simulink model "STOICAL_example_1"  (R2015b)
settings: Solver=ode4  StartTime=0.0  StopTime=1  FixedStep=50E-6  RelTol=1e-3
model workspace (MAT data in the model file):
  STOICAL.SignalSaveOptions.ReturnWorkspaceOutputs = 'on'
  STOICAL.SignalSaveOptions.ReturnWorkspaceOutputsName = 'simout_obj'
  STOICAL.SignalSaveOptions.SignalLogging = 'on'
  STOICAL.SignalSaveOptions.SignalLoggingSaveFormat = 'Dataset'
  STOICAL.SignalSaveOptions.SignalLoggingName = 'STOVICAL_LoggedSignals'
  STOICAL.ParameterDefinition.BlkNameFull{1} = 'Step amplitude
    | #PARAM#Amplitude'
  STOICAL.ParameterDefinition.BlkNameFull{2} = 'Static System
    | modelled
    | by gain block
    | #PARAM#SystemGain'
  STOICAL.ParameterDefinition.BlkNameShort{1} = 'Step amplitude
    | '
  STOICAL.ParameterDefinition.BlkNameShort{2} = 'Static System
    | modelled
    | by gain block
    | '
  STOICAL.ParameterDefinition.BlkHandle = [1972.00012207; 1979.00012207]
  STOICAL.ParameterDefinition.ParamName = {'Amplitude'; 'SystemGain'}
  STOICAL.ParameterDefinition.BlkPath{1} = 'STOICAL_example_1_Step02b_ActivateParameters/#UNIT#Stimulus/Step amplitude
    | #PARAM#Amplitude'
  STOICAL.ParameterDefinition.BlkPath{2} = 'STOICAL_example_1_Step02b_ActivateParameters/#UNIT#System/Static System
    | modelled
    | by gain block
    | #PARAM#SystemGain'
  STOICAL.ParameterDefinition.BlkType = {'Constant'; 'Gain'}
  STOICAL.ParameterDefinition.BlkMaskType = {''; ''}
  STOICAL.ParameterDefinition.ParentalBlockPath = {'STOICAL_example_1_Step02b_ActivateParameters/#UNIT#Stimulus'; 'STOICAL_example_1_Step02b_ActivateParameters/#UNIT#System'}
  STOICAL.ParameterDefinition.ParentalBlockHandle = [1969.00012207; 1977.00036621]
  STOICAL.ParameterDefinition.Belongs2SubsystemHdl = [1969.00012207; 1977.00036621]
  STOICAL.ParameterDefinition.NrParams = 2
  STOICAL.ParameterDefinition.BlkField2Set = {'Value'; 'Gain'}
  STOICAL.ParameterDefinition.BlkFieldSyntax = {'#'; '#'}
  STOICAL.ParameterDefinition.ParamVariable = {'param_ec6e274da2c23e664dfdc874ac252818'; 'param_afc1e04cc1c158b687408e5b6ea19d06'}
  STOICAL.ParameterDefinition.LabelPath = {'#Stimulus#Amplitude'; '#System#SystemGain'}
  STOICAL.ParameterDefinition.ParamDefaultValue = {'2'; '5'}
  STOICAL.SignalDefinition.ParentalBlockPath = {'STOICAL_example_1_Step02c_ActivateSignals'; 'STOICAL_example_1_Step02c_ActivateSignals'}
  STOICAL.SignalDefinition.ParentalBlockHandle = [1967.00048828; 1967.00048828]
  STOICAL.SignalDefinition.NameInDiagram = {'#SIG#stimulus'; '#SIG#response'}
  STOICAL.SignalDefinition.SourceBlockPath = {'STOICAL_example_1_Step02c_ActivateSignals/#UNIT#Stimulus'; 'STOICAL_example_1_Step02c_ActivateSignals/#UNIT#System'}
  STOICAL.SignalDefinition.SourceBlockPort = [1; 1]
  STOICAL.SignalDefinition.SourceBlockHandle = [1969.00195312; 1977.00073242]
  STOICAL.SignalDefinition.Handle = [1988.00097656; 1989.00073242]
  STOICAL.SignalDefinition.NrSig = 2
  STOICAL.SignalDefinition.NameOfLogVar = {'logsig_47c2411a71c8218b6c2a20514199b03d'; 'logsig_5069e1d9063564028bd2189e4cf0bc84'}
  STOICAL.SignalDefinition.NameOfLogVarMode = {'SignalName'; 'SignalName'}
  STOICAL.SignalDefinition.DoLog = [0; 0]
  STOICAL.SignalDefinition.LabelPath = {'#stimulus'; '#response'}
  STOICAL.VariantDefinition.NodeHandle = [1967.00073242; 1969.00561523; 1977.00146484]
  STOICAL.VariantDefinition.NodeName = {'STOICAL_example_1_Step02d_ActivateVariants'; '#UNIT#Stimulus'; '#UNIT#System'}
  STOICAL.VariantDefinition.IsVariantSubsystem = [0; 0; 0]
  STOICAL.VariantDefinition.NodeLevel = [1; 2; 2]
  STOICAL.VariantDefinition.NodePath = {'STOICAL_example_1_Step02d_ActivateVariants'; 'STOICAL_example_1_Step02d_ActivateVariants/#UNIT#Stimulus'; 'STOICAL_example_1_Step02d_ActivateVariants/#UNIT#System'}
  STOICAL.VariantDefinition.IsVariant = [0; 0; 0]
  STOICAL.VariantDefinition.VSNodeIdxofVariant = [0; 0; 0]
  STOICAL.VariantDefinition.VSVariantsCount = [0; 0; 0]
  STOICAL.VariantDefinition.VSVariantsBlkHdls = {[]; []; []}
  STOICAL.VariantDefinition.VSVariantsNodeIdx = {[]; []; []}
  STOICAL.VariantDefinition.VSControlVariable = {[]; []; []}
  STOICAL.VariantDefinition.VSVariantHasNr = [0; 0; 0]
  STOICAL.VariantDefinition.LabelPath = {[]; []; []}
  param_afc1e04cc1c158b687408e5b6ea19d06 = '5'
  param_ec6e274da2c23e664dfdc874ac252818 = '2'
settings Model: Creator=Wippenbeck  LastModifiedBy=bertram
settings DataIOCC: SaveFormat=Array  ReturnWorkspaceOutputs=on  SignalLoggingName=STOVICAL_LoggedSignals  ReturnWorkspaceOutputsName=simout_obj
settings DebuggingCC: SolverPrmCheckMsg=warning
settings HardwareCC: ProdBitPerPointer=32  ProdLargestAtomicFloat=None  ProdIntDivRoundTo=Undefined  ProdEndianess=Unspecified  ProdWordSize=32  ProdHWDeviceType=32-bit Generic
settings GRTTargetCC: GeneratePreprocessorConditionals=Disable all
settings ConfigComp: CovModelRefEnable=Off  CovSFcnEnable=off

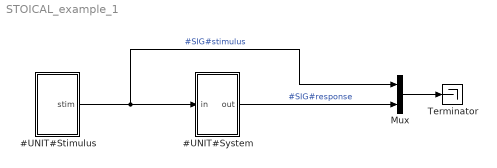
== system STOICAL_example_1 ==
  #UNIT#Stimulus : Subsystem
  #UNIT#System : Subsystem
  Mux : Mux  Inputs=2
  Terminator : Terminator
  wires:
  Mux/1 -> Terminator/1
  #UNIT#Stimulus/1(stim) -> #UNIT#System/1(in), Mux/1  "#SIG#stimulus"
  #UNIT#System/1(out) -> Mux/2  "#SIG#response"

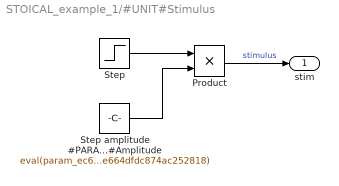
== system STOICAL_example_1/#UNIT#Stimulus ==
  Product : Product
  Step : Step  Time=0.1  SampleTime=0
  Step amplitude #PARAM#Amplitude : Constant  Value=eval(param_ec6e274da2c23e664dfdc874ac252818)
  stim : Outport
  wires:
  Step amplitude #PARAM#Amplitude/1 -> Product/2
  Product/1 -> stim/1  "stimulus"
  Step/1 -> Product/1

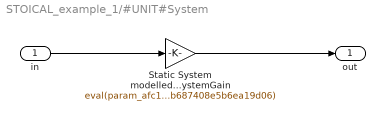
== system STOICAL_example_1/#UNIT#System ==
  in : Inport
  Static System modelled by gain block #PARAM#SystemGain : Gain  Gain=eval(param_afc1e04cc1c158b687408e5b6ea19d06)
  out : Outport
  wires:
  Static System modelled by gain block #PARAM#SystemGain/1 -> out/1
  in/1 -> Static System modelled by gain block #PARAM#SystemGain/1
